simulink library "waijung_image_sensor_lib"  (R2015b)
settings: Solver=ode45  StartTime=0.0  StopTime=10.0  RelTol=1e-3
libraries: simulink x11, stm32f4_i2c_lib x8, stm32f4_tim_lib x2
settings Model: Creator=Krisada  LastModifiedBy=Aimagin
settings DataIOCC: SaveFormat=Array  SignalLoggingSaveFormat=ModelDataLogs
settings OptimizationCC: ExpressionDepthLimit=2147483647
settings DebuggingCC: UnderspecifiedInitializationDetection=Classic  MergeDetectMultiDrivingBlocksExec=none  SolverPrmCheckMsg=warning  FcnCallInpInsideContextMsg=UseLocalSettings  StateNameClashWarn=warning  StrictBusMsg=Warning
settings HardwareCC: ProdBitPerPointer=32  ProdLargestAtomicFloat=None  ProdIntDivRoundTo=Undefined  ProdEndianess=Unspecified  ProdWordSize=32  ProdHWDeviceType=32-bit Generic
settings GRTTargetCC: CombineOutputUpdateFcns=off  GRTInterface=on
settings ConfigComp: CovModelRefEnable=Off

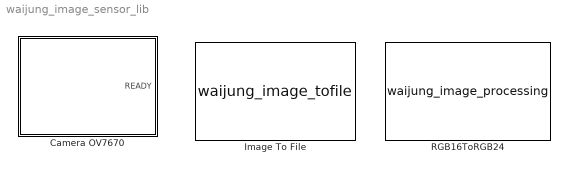
== system waijung_image_sensor_lib ==
  Camera OV7670 : Subsystem  mask{camera=OV7670, storagename=ExtRAM, xclkfreq=8MHz(MCO), imgsize=120 x 160, module=1, slvaddr=hex2dec('42'), sampletime=-1}
      mask prompts: storagename "Output buffer"; xclkfreq "XCLK input frequency"; imgsize "Image size"; module "I2C Module"; slvaddr "I2C Slave address"; sampletime "Sample time (sec)"
      mask init:
      | waijung_image_sensor_callback('init');
      mask TypeOptions camera: OV7670
      mask Callback camera: waijung_image_sensor_callback('camera');
      mask TypeOptions storagename: ExtRAM
      mask Callback storagename: waijung_image_sensor_callback('storagename');
      mask TypeOptions xclkfreq: 8MHz(MCO) | 24MHz
      mask TypeOptions imgsize: 120 x 160 | 240 x 320 | 480 x 640
      mask TypeOptions module: 1 | 2 | 3
      mask Callback module: waijung_image_sensor_callback('module');
      mask Display: text(0.5, 0.5, '[OV7670]\nPort: I2C1','ver','middle','hor','center');port_label('output', 1,'READY');
  Image To File : S-Function  FunctionName=waijung_image_tofile  Parameters=conf,inputporttype,inputportwidth,outputporttype,outputportwidth,optionstring,sampletime,blockid  SFunctionDeploymentMode=off  EnableBusSupport=off  mask(waijung_image_tofile){conf=ToFile, variablefilename=on, filename=Image.bmp, format=BMP, size=QQVGA (160 x 120), storagename=<Manual Configure>, varname=0x64000000, storagetype=uint16, storagesize=160*120*2, portpinstr=0, rgb16torgb24=on, enablestatus=on, sampletime=-1, blockid=ImageToFile, inputporttype=[7], inputportwidth=[], inputportlabel={'Filename'}, outputporttype=[7], outputportwidth=[], outputportlabel={'Status'}, compat=0, optionstring=[]}
      mask prompts: conf "Configuration"; variablefilename "Variable file name"; filename "File name"; storagename "Source buffer"; varname "Source buffer var name"; storagetype "Source buffer var type"; storagesize "Source buffer size"; portpinstr "Port Pin String"; rgb16torgb24 "Enable RGB16 to RGB24 conversion"; enablestatus "Enable output status"; sampletime "Sample time (sec)"; blockid "Block ID"; inputporttype "Input Port Type"; inputportwidth "Input Port Width"; inputportlabel "Input Port Label"; outputporttype "Output Port Type"; outputportwidth "Output Port Width"; outputportlabel "Output port label"; compat "Compatibility (Reserved for future use)"; optionstring "String(s) to be passed to TLC"
      mask init:
      | waijung_image_tofile_callback('init');
      mask Help: web(fullfile(waijungdocroot,'waijung_image_tofile.htm'), '-browser')
      mask TypeOptions conf: ToFile
      mask Callback conf: waijung_image_tofile_callback('conf');
      mask Callback variablefilename: waijung_image_tofile_callback('variablefilename');
      mask TypeOptions format: BMP | JPG
      mask TypeOptions size: QQVGA (160 x 120) | QVGA (320 x 240) | VGA (640 x 480)
      mask TypeOptions storagename: <Manual Configure>
      mask Callback storagename: stm32f4_dcmi_callback('storagename');
      mask TypeOptions storagetype: double | single | int8 | uint8 | int16 | uint16 | int32 | uint32
      mask Callback enablestatus: waijung_image_tofile_callback('enablestatus');
      mask Callback sampletime: waijung_image_tofile_callback('sampletime');
      mask Callback blockid: waijung_image_tofile_callback('blockid');
      mask Display: text(0.5, 0.5, '[ BMP ]\nQQVGA (160 x 120)','ver','middle','hor','center'); port_label('input', 1,'Filename'); port_label('output', 1,'Status');
  RGB16ToRGB24 : S-Function  FunctionName=waijung_image_processing  Parameters=conf,inputporttype,inputportwidth,outputporttype,outputportwidth,row,column,optionstring,simparams,sampletime,blockid  SFunctionDeploymentMode=off  EnableBusSupport=off  mask(waijung_image_processing){conf=RGB16ToRGB24, column=10, row=10, inputalignment=RGB, outputalignment=RGB, colorseparate=on, simparams=[0 10 0 0], portpinstr=0, sampletime=-1, blockid=RGB16ToRGB24, inputporttype=[5], inputportwidth=[100], inputportlabel={'Input'}, outputporttype=[3  3 3], outputportwidth=[10 10 10], outputportlabel={'R','G','B'}, compat=0, optionstring=[]}
      mask prompts: conf "Configuration"; column "Image width (Column, M)"; row "Image heigh (Row, N)"; inputalignment "Input color alignment"; outputalignment "Output color alignment"; colorseparate "Separate output color"; simparams "Simulate params"; portpinstr "Port Pin String"; sampletime "Sample time (sec)"; blockid "Block ID"; inputporttype "Input Port Type"; inputportwidth "Input Port Width"; inputportlabel "Input Port Label"; outputporttype "Output Port Type"; outputportwidth "Output Port Width"; outputportlabel "Output port label"; compat "Compatibility (Reserved for future use)"; optionstring "String(s) to be passed to TLC"
      mask help: RGB16: R(5)-G(6)-B(5)
      mask init:
      | waijung_image_processing_callback('init');
      mask Help: web(fullfile(waijungdocroot,'waijung_image_processing.htm'), '-browser')
      mask TypeOptions conf: RGB16ToRGB24
      mask Callback conf: waijung_image_processing_callback('conf');
      mask Callback column: waijung_image_processing_callback('updateport');
      mask TypeOptions inputalignment: RGB | BGR
      mask Callback inputalignment: waijung_image_processing_callback('updateport');
      mask TypeOptions outputalignment: RGB | BGR
      mask Callback outputalignment: waijung_image_processing_callback('updateport');
      mask Callback colorseparate: waijung_image_processing_callback('updateport');
      mask Callback sampletime: waijung_image_processing_callback('sampletime');
      mask Callback blockid: waijung_image_processing_callback('blockid');
      mask Display: text(0.5, 0.5, '[RGB16ToRGB24]','ver','middle','hor','center'); port_label('input', 1,'Input'); port_label('output', 1,'R'); port_label('output', 2,'G'); port_label('output', 3,'B');

== system waijung_image_sensor_lib/Camera OV7670 ==
  Capture_ : Subsystem  TreatAsAtomicUnit=on
  Init_ : Subsystem
  Logical Operator : Logic  Operator=NOT  AllPortsSameDT=off  OutDataTypeStr=boolean
  Memory : Memory  InheritSampleTime=on
  Rate Transition : RateTransition  OutPortSampleTime=sampletime
  READY : Outport
  wires:
  Capture_/1(SUCCESS) -> READY/1
  Init_/1(Out1) -> Memory/1
  Memory/1 -> Logical Operator/1, Rate Transition/1
  Logical Operator/1 -> Init_/Enable
  Rate Transition/1 -> Capture_/Enable

== system waijung_image_sensor_lib/Camera OV7670/Capture_ ==
  Enable : EnablePort  PropagateVarSize=During execution
  Compare To Zero : simulink/Logic and Bit Operations/Compare To Zero  SystemSampleTime=-1  relop===  LogicOutDataTypeMode=uint8  ZeroCross=off
  DCMI Capture : S-Function  FunctionName=stm32f4_dcmi  Parameters=conf,inputporttype,inputportwidth,outputporttype,outputportwidth,optionstring,sampletime,blockid  SFunctionDeploymentMode=off  EnableBusSupport=off  mask(stm32f4_dcmi){conf=DCMI, capturemode=SnapShot, synchronizemode=Hardware, pclkpolarity=Falling, vspolarity=High, hspolarity=High, capturerate=All, capturesize=120*160*2, storagename=<Manual Configure>, varname=VolatileDataArray_ExtRAM, storagetype=uint16, storagesize=120*160, remap=Profile #2, sampletime=inf, blockid=CameraOV7670Capture_DCMICapture, inputporttype=[], inputportwidth=[], inputportlabel={}, outputporttype=[7], outputportwidth=[], outputportlabel={'Status'}, compat=0, optionstring=["DCMI","SnapShot","Hardware","Falling","High","High","All","0","Word","9600","0","0","VolatileDataArray_ExtRAM"," "," "," ","1","0","0","0","0","0","0","1","1","A","6","I","5","H","8","H","9","H","10","H","11","H","12","H","14","I","4","I","6","I","7"], portpinstr=A6,I5,H8,H9,H10,H11,H12,H14,I4,I6,I7}
      mask prompts: conf "Configuration"; capturemode "Capture mode"; synchronizemode "Synchronization Mode"; pclkpolarity "Pixel clock polarity"; vspolarity "Vertical synchronization polarity"; hspolarity "Horizontal synchronization polarity"; capturerate "Capture rate"; capturesize "Capture data size (Bytes)"; storagename "Output buffer"; varname "Output buffer var name"; storagetype "Output buffer var type"; storagesize "Output buffer size (Total bytes must be equal to, or greater than DMA Transfer size)"; remap "Remap DCMI pins"; sampletime "Sample time (sec)"; inputporttype "Input port"; inputportwidth "Input Port Width"; inputportlabel "Input port label"; outputporttype "Output port"; outputportwidth "Output Port Width"; outputportlabel "Output port label"; compat "Compatibility (Reserved for future use)"; optionstring "Configuration String"; portpinstr "Port Pin String"
      mask help:
      | Synchronize mode:
      |  - Hardware: Hardware synchronization data capture is synchronized with the HSYNC/VSYNC signals.
      |  - Embedded: Embedded synchronization data capture is synchronized with synchronization codes embedded in the data flow.
      | Pixel clock polarity:
      |  - Falling: Pixel clock active on Falling edge.
      |  - Rising: Pixel clock active on Rising edge.
      | Vertical, Horizontal sychronization polarity:
      |  - Low: vertical synchronization active Low.
      |  - High: Vertical synchronization active High.
      | Capture rate:
      |  - All: All frames are captured.
      |  - 1of2: Every alternate frame captured.
      |  - 1of4: On frame in 4 frames captured.
      | Pins Profile:
      | Set of configuration pins for: PIXCLK, VSYNC, HSYNC, D0, D1, .., D7 corresponding.
      |  - Profile #1: PA6, PB7, PA4, PC6, PC7,  PE0,  PE1,  PE4,  PB6, PE5, PE6
      |  - Profile #2: PA6, PI5, PH8, PH9, PH10, PH11, PH12, PH14, PI4, PI6, PI7
      mask init:
      | stm32f4_dcmi_callback('init');
      mask Help: web(fullfile(waijungdocroot,'stm32f4_dcmi.htm'), '-browser')
      mask TypeOptions conf: DCMI
      mask Callback conf: stm32f4_dcmi_callback('conf');
      mask TypeOptions capturemode: Continuous | SnapShot
      mask TypeOptions synchronizemode: Hardware | Embedded
      mask TypeOptions pclkpolarity: Falling | Rising
      mask TypeOptions vspolarity: High | Low
      mask TypeOptions hspolarity: High | Low
      mask TypeOptions capturerate: All | 1of2 | 1of4
      mask TypeOptions storagename: <Manual Configure>
      mask Callback storagename: stm32f4_dcmi_callback('storagename');
      mask TypeOptions storagetype: double | single | int8 | uint8 | int16 | uint16 | int32 | uint32
      mask Callback storagesize: stm32f4_dcmi_callback('storagesize');
      mask TypeOptions remap: Profile #1 | Profile #2
      mask Callback remap: stm32f4_dcmi_callback('remap');
      mask Callback sampletime: stm32f4_dcmi_callback('sampletime');
      mask Callback blockid: stm32f4_dcmi_callback('blockid');
      mask Display: text(0.05, 0.5, 'Size: 38400\nPins: Profile #2\nTs (sec): 0','ver','middle','hor','left'); port_label('output', 1,'Status');
  SUCCESS : Outport
  wires:
  Compare To Zero/1 -> SUCCESS/1
  DCMI Capture/1 -> Compare To Zero/1

== system waijung_image_sensor_lib/Camera OV7670/Init_ ==
  Enable : EnablePort  PropagateVarSize=During execution
  While Iterator_ : Subsystem  TreatAsAtomicUnit=on
  Out1 : Outport
  wires:
  While Iterator_/1(Ready) -> Out1/1

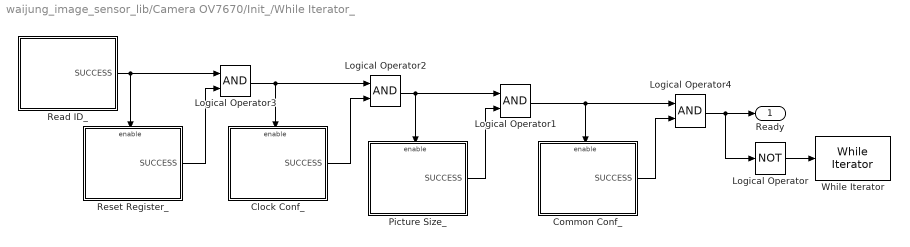
== system waijung_image_sensor_lib/Camera OV7670/Init_/While Iterator_ ==
  Clock Conf_ : Subsystem
  Common Conf_ : Subsystem
  Logical Operator : Logic  Operator=NOT  AllPortsSameDT=off  OutDataTypeStr=boolean
  Logical Operator{1..4} (4 alike) : Logic  AllPortsSameDT=off  OutDataTypeStr=boolean
  Picture Size_ : Subsystem
  Read ID_ : Subsystem
  Reset Register_ : Subsystem
  While Iterator : WhileIterator  MaxIters=-1  WhileBlockType=do-while
  Ready : Outport
  wires:
  Logical Operator3/1 -> Clock Conf_/Enable, Logical Operator2/1
  Read ID_/1(SUCCESS) -> Reset Register_/Enable, Logical Operator3/1
  Picture Size_/1(SUCCESS) -> Logical Operator1/2
  Logical Operator1/1 -> Common Conf_/Enable, Logical Operator4/1
  Logical Operator/1 -> While Iterator/1
  Reset Register_/1(SUCCESS) -> Logical Operator3/2
  Clock Conf_/1(SUCCESS) -> Logical Operator2/2
  Logical Operator2/1 -> Logical Operator1/1, Picture Size_/Enable
  Logical Operator4/1 -> Logical Operator/1, Ready/1
  Common Conf_/1(SUCCESS) -> Logical Operator4/2

== system waijung_image_sensor_lib/Camera OV7670/Init_/While Iterator_/Clock Conf_ ==
  Enable : EnablePort  PropagateVarSize=During execution
  Logical Operator : Logic  Operator=NOT  AllPortsSameDT=off  OutDataTypeStr=boolean
  Memory : Memory  InheritSampleTime=on
  Subsystem : Subsystem
  SUCCESS : Outport
  wires:
  Memory/1 -> Logical Operator/1
  Logical Operator/1 -> Subsystem/Enable
  Subsystem/1(Out1) -> Memory/1, SUCCESS/1

== system waijung_image_sensor_lib/Camera OV7670/Init_/While Iterator_/Common Conf_ ==
  Enable : EnablePort  PropagateVarSize=During execution
  Logical Operator : Logic  Operator=NOT  AllPortsSameDT=off  OutDataTypeStr=boolean
  Memory : Memory  InheritSampleTime=on
  Subsystem : Subsystem
  SUCCESS : Outport
  wires:
  Memory/1 -> Logical Operator/1
  Logical Operator/1 -> Subsystem/Enable
  Subsystem/1(Out1) -> Memory/1, SUCCESS/1

== system waijung_image_sensor_lib/Camera OV7670/Init_/While Iterator_/Picture Size_ ==
  Enable : EnablePort  PropagateVarSize=During execution
  Logical Operator : Logic  Operator=NOT  AllPortsSameDT=off  OutDataTypeStr=boolean
  Memory : Memory  InheritSampleTime=on
  Subsystem : Subsystem
  SUCCESS : Outport
  wires:
  Subsystem/1(Out1) -> SUCCESS/1, Memory/1
  Logical Operator/1 -> Subsystem/Enable
  Memory/1 -> Logical Operator/1

== system waijung_image_sensor_lib/Camera OV7670/Init_/While Iterator_/Read ID_ ==
  Logical Operator : Logic  Operator=NOT  AllPortsSameDT=off  OutDataTypeStr=boolean
  Memory : Memory  InheritSampleTime=on
  Subsystem_ : Subsystem
  SUCCESS : Outport
  wires:
  Subsystem_/1(Out1) -> SUCCESS/1, Memory/1
  Logical Operator/1 -> Subsystem_/Enable
  Memory/1 -> Logical Operator/1

== system waijung_image_sensor_lib/Camera OV7670/Init_/While Iterator_/Reset Register_ ==
  Enable : EnablePort  PropagateVarSize=During execution
  Logical Operator : Logic  Operator=NOT  AllPortsSameDT=off  OutDataTypeStr=boolean
  Memory : Memory  InheritSampleTime=on
  Subsystem : Subsystem
  SUCCESS : Outport
  wires:
  Memory/1 -> Logical Operator/1
  Logical Operator/1 -> Subsystem/Enable
  Subsystem/1(Out1) -> Memory/1, SUCCESS/1

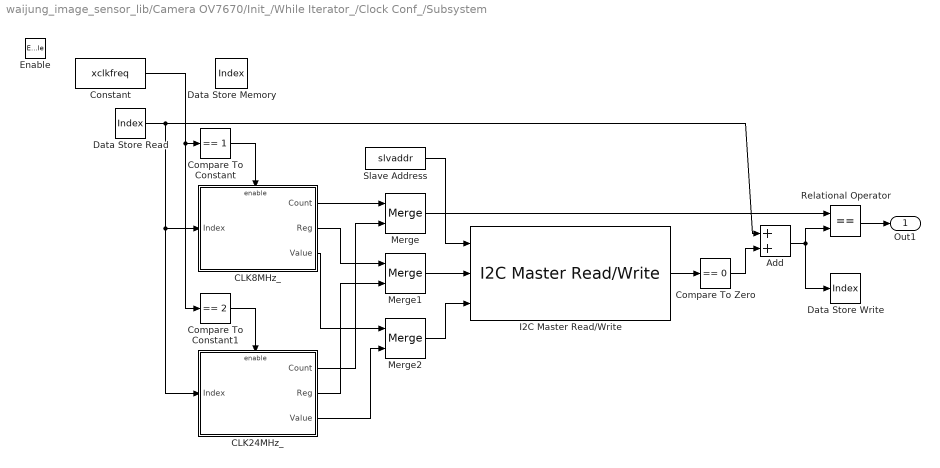
== system waijung_image_sensor_lib/Camera OV7670/Init_/While Iterator_/Clock Conf_/Subsystem ==
  Enable : EnablePort  PropagateVarSize=During execution
  Add : Sum
  CLK24MHz_ : Subsystem  TreatAsAtomicUnit=on
  CLK8MHz_ : Subsystem  TreatAsAtomicUnit=on
  Compare To Constant : simulink/Logic and Bit Operations/Compare To Constant  SystemSampleTime=-1  relop===  const=1  LogicOutDataTypeMode=boolean  ZeroCross=off
  Compare To Constant1 : simulink/Logic and Bit Operations/Compare To Constant  SystemSampleTime=-1  relop===  const=2  LogicOutDataTypeMode=boolean  ZeroCross=off
  Compare To Zero : simulink/Logic and Bit Operations/Compare To Zero  SystemSampleTime=-1  relop===  LogicOutDataTypeMode=uint8  ZeroCross=off
  Constant : Constant  Value=xclkfreq
  Data Store Memory : DataStoreMemory  DataStoreName=Index  ReadBeforeWriteMsg=warning  WriteAfterWriteMsg=warning  WriteAfterReadMsg=warning  OutDataTypeStr=uint8
  Data Store Read : DataStoreRead  DataStoreName=Index
  Data Store Write : DataStoreWrite  DataStoreName=Index
  I2C Master Read/Write : stm32f4_i2c_lib/I2C Master Read//Write  configuration=Transaction  module=1  lastmodule=3  transfer=Blocking  dutycycle=TLow/THigh = 2  clkspeed=400  timeout=25  writecount=2  readcount=0  sdapin=C9  sclpin=A8  waitwritetime=5  forcestop=off  inputtypearray=[3 3 3 3]  outputtypearray=[1 3]  confstr="[\"C\",\"9\",\"A\",\"8\",\"1\",\"1\",\"6\",\"0\",\"I2C_DutyCycle_2\",\"5\",\"off\"]"  sampletime=-1  sampletimestr=-1  blockid=CameraOV1Init_WhileIterator_ClockConf_SubsystemI2CMasterReadWrite
  Merge : Merge
  Merge1 : Merge
  Merge2 : Merge
  Relational Operator : RelationalOperator  Operator===  OutDataTypeStr=boolean
  Slave Address : Constant  Value=slvaddr  OutDataTypeStr=uint8
  Out1 : Outport
  wires:
  Relational Operator/1 -> Out1/1
  Add/1 -> Data Store Write/1, Relational Operator/2
  Compare To Zero/1 -> Add/2
  I2C Master Read/Write/1 -> Compare To Zero/1
  Data Store Read/1 -> Add/1, CLK8MHz_/1(Index), CLK24MHz_/1(Index)
  Slave Address/1 -> I2C Master Read/Write/1
  Compare To Constant/1 -> CLK8MHz_/Enable
  Compare To Constant1/1 -> CLK24MHz_/Enable
  CLK8MHz_/1(Count) -> Merge/1
  CLK8MHz_/2(Reg) -> Merge1/1
  CLK8MHz_/3(Value) -> Merge2/1
  CLK24MHz_/1(Count) -> Merge/2
  CLK24MHz_/2(Reg) -> Merge1/2
  CLK24MHz_/3(Value) -> Merge2/2
  Constant/1 -> Compare To Constant/1, Compare To Constant1/1
  Merge/1 -> Relational Operator/1
  Merge1/1 -> I2C Master Read/Write/2
  Merge2/1 -> I2C Master Read/Write/3

== system waijung_image_sensor_lib/Camera OV7670/Init_/While Iterator_/Common Conf_/Subsystem ==
  Enable : EnablePort  PropagateVarSize=During execution
  Add : Sum
  Compare To Zero : simulink/Logic and Bit Operations/Compare To Zero  SystemSampleTime=-1  relop===  LogicOutDataTypeMode=uint8  ZeroCross=off
  Data Store Memory : DataStoreMemory  DataStoreName=Index  ReadBeforeWriteMsg=warning  WriteAfterWriteMsg=warning  WriteAfterReadMsg=warning  OutDataTypeStr=uint8
  Data Store Read : DataStoreRead  DataStoreName=Index
  Data Store Write : DataStoreWrite  DataStoreName=Index
  I2C Master Read/Write : stm32f4_i2c_lib/I2C Master Read//Write  configuration=Transaction  module=1  lastmodule=3  transfer=Blocking  dutycycle=TLow/THigh = 2  clkspeed=400  timeout=25  writecount=2  readcount=0  sdapin=C9  sclpin=A8  waitwritetime=5  forcestop=off  inputtypearray=[3 3 3 3]  outputtypearray=[1 3]  confstr="[\"C\",\"9\",\"A\",\"8\",\"1\",\"1\",\"6\",\"0\",\"I2C_DutyCycle_2\",\"5\",\"off\"]"  sampletime=-1  sampletimestr=-1  blockid=CameraOV1Init_WhileIterator_CommonConf_SubsystemI2CMasterReadWrite
  Register List : Subsystem  mask{register=uint8([122,123,124,125,126,127,128,129,130,131,132,133,134,135,136,137,19,21,0,16,13,20,165,171,36,37,38,159,160,161,166,167,168,169,170,19,14,15,22,30,33,34,41,51,53,55,56,57,60,77,78,105,116,141,142,143,144,145,146,150,154,176,177,178,179,184,67,68,69,70,71,72,89,90,91,92,93,94,100,101,102,148,149,108,109,110,111,106,1,2,19,21,79,80,81,82,83,84,85,86,87,88,65,63,117,118,76,119,75,201,65,86,52,59,164,150,157,158,9,59]), value=uint8([32,28,40,60,85,104,118,128,136,143,150,163,175,196,215,232,232,24,15,0,0,32,5,7,117,99,165,120,104,3,223,223,240,144,148,229,97,75,2,39,2,145,7,11,11,29,113,42,120,64,32,0,25,79,0,0,0,0,0,0,128,132,12,14,130,10,20,240,52,88,40,58,136,136,68,103,73,14,4,32,5,4,8,10,85,17,159,64,64,64,231,24,128,128,0,34,94,128,0,82,128,158,8,5,5,225,15,10,9,192,56,64,17,2,137,0,76,63,2,66])}
      mask prompts: register "Register Index"; value "Register Value"
      mask help:
      | Count:
      |  - Number of Register-Value pair.
      |  - Determine from lowest size, between Register and Value.
      | Reg:
      |  - Register index.
      | Value:
      |  - Data corresponding to specified register index.
  Relational Operator : RelationalOperator  Operator===  OutDataTypeStr=boolean
  Slave Address : Constant  Value=slvaddr  OutDataTypeStr=uint8
  Out1 : Outport
  wires:
  Register List/1(Count) -> Relational Operator/1
  Register List/3(Value) -> I2C Master Read/Write/3
  Register List/2(Reg) -> I2C Master Read/Write/2
  Relational Operator/1 -> Out1/1
  Add/1 -> Data Store Write/1, Relational Operator/2
  Compare To Zero/1 -> Add/2
  I2C Master Read/Write/1 -> Compare To Zero/1
  Data Store Read/1 -> Register List/1(Index), Add/1
  Slave Address/1 -> I2C Master Read/Write/1

== system waijung_image_sensor_lib/Camera OV7670/Init_/While Iterator_/Picture Size_/Subsystem ==
  Enable : EnablePort  PropagateVarSize=During execution
  Add : Sum
  Compare To Zero : simulink/Logic and Bit Operations/Compare To Zero  SystemSampleTime=-1  relop===  LogicOutDataTypeMode=uint8  ZeroCross=off
  Data Store Memory : DataStoreMemory  DataStoreName=Index  ReadBeforeWriteMsg=warning  WriteAfterWriteMsg=warning  WriteAfterReadMsg=warning  OutDataTypeStr=uint8
  Data Store Read : DataStoreRead  DataStoreName=Index
  Data Store Write : DataStoreWrite  DataStoreName=Index
  I2C Master Read/Write : stm32f4_i2c_lib/I2C Master Read//Write  configuration=Transaction  module=1  lastmodule=3  transfer=Blocking  dutycycle=TLow/THigh = 2  clkspeed=400  timeout=25  writecount=2  readcount=0  sdapin=C9  sclpin=A8  waitwritetime=5  forcestop=off  inputtypearray=[3 3 3 3]  outputtypearray=[1 3]  confstr="[\"C\",\"9\",\"A\",\"8\",\"1\",\"1\",\"6\",\"0\",\"I2C_DutyCycle_2\",\"5\",\"off\"]"  sampletime=-1  sampletimestr=-1  blockid=CameraOV1Init_WhileIterator_PictureSize_SubsystemI2CMasterReadWrite
  Relational Operator : RelationalOperator  Operator===  OutDataTypeStr=boolean
  Slave Address : Constant  Value=slvaddr  OutDataTypeStr=uint8
  Subsystem : Subsystem
  Out1 : Outport
  wires:
  Slave Address/1 -> I2C Master Read/Write/1
  Data Store Read/1 -> Add/1, Subsystem/1(Index)
  I2C Master Read/Write/1 -> Compare To Zero/1
  Compare To Zero/1 -> Add/2
  Add/1 -> Relational Operator/2, Data Store Write/1
  Relational Operator/1 -> Out1/1
  Subsystem/3(Value) -> I2C Master Read/Write/3
  Subsystem/2(Reg) -> I2C Master Read/Write/2
  Subsystem/1(Count) -> Relational Operator/1

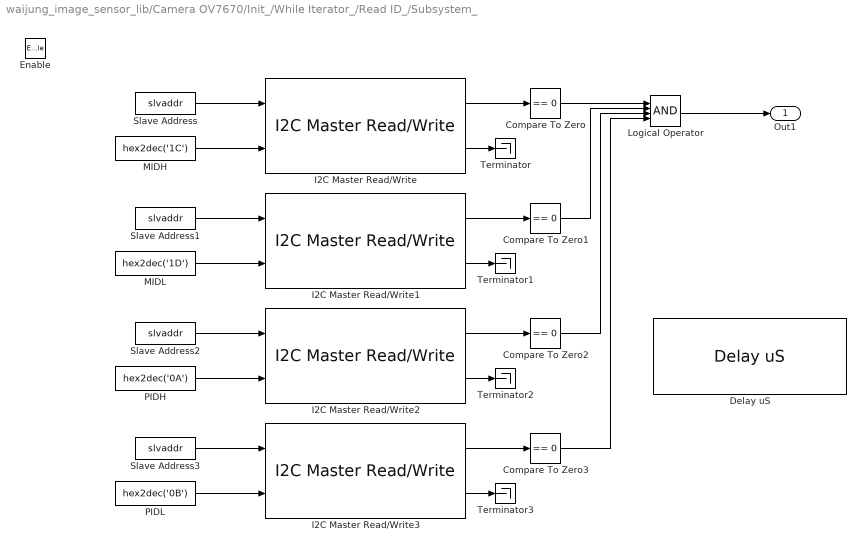
== system waijung_image_sensor_lib/Camera OV7670/Init_/While Iterator_/Read ID_/Subsystem_ ==
  Enable : EnablePort  PropagateVarSize=During execution
  Compare To Zero{,1..3} (4 alike) : simulink/Logic and Bit Operations/Compare To Zero  SystemSampleTime=-1  relop===  LogicOutDataTypeMode=uint8  ZeroCross=off
  Delay uS : stm32f4_tim_lib/Delay uS  Priority=0  delaytime=300000  enableinput=off  enableoutput=off  inputtypearray=[0]  outputtypearray=[0]  sampletime=-1  sampletimestr=-1  blockid=CameraOV1Init_WhileIterator_ReadID_Subsystem_DelayuS
  I2C Master Read/Write : stm32f4_i2c_lib/I2C Master Read//Write  configuration=Transaction  module=1  lastmodule=3  transfer=Blocking  dutycycle=TLow/THigh = 2  clkspeed=400  timeout=25  writecount=1  readcount=1  sdapin=C9  sclpin=A8  waitwritetime=0  forcestop=on  inputtypearray=[2 3 3]  outputtypearray=[2 3 3]  confstr="[\"C\",\"9\",\"A\",\"8\",\"1\",\"1\",\"6\",\"0\",\"I2C_DutyCycle_2\",\"0\",\"on\"]"  sampletime=-1  sampletimestr=-1  blockid=CameraOV1Init_WhileIterator_ReadID_Subsystem_I2CMasterReadWrite
  I2C Master Read/Write1 : stm32f4_i2c_lib/I2C Master Read//Write  configuration=Transaction  module=1  lastmodule=3  transfer=Blocking  dutycycle=TLow/THigh = 2  clkspeed=400  timeout=25  writecount=1  readcount=1  sdapin=C9  sclpin=A8  waitwritetime=0  forcestop=on  inputtypearray=[2 3 3]  outputtypearray=[2 3 3]  confstr="[\"C\",\"9\",\"A\",\"8\",\"1\",\"1\",\"6\",\"0\",\"I2C_DutyCycle_2\",\"0\",\"on\"]"  sampletime=-1  sampletimestr=-1  blockid=CameraOV1Init_WhileIterator_ReadID_Subsystem_I2CMasterReadWrite1
  I2C Master Read/Write2 : stm32f4_i2c_lib/I2C Master Read//Write  configuration=Transaction  module=1  lastmodule=3  transfer=Blocking  dutycycle=TLow/THigh = 2  clkspeed=400  timeout=25  writecount=1  readcount=1  sdapin=C9  sclpin=A8  waitwritetime=0  forcestop=on  inputtypearray=[2 3 3]  outputtypearray=[2 3 3]  confstr="[\"C\",\"9\",\"A\",\"8\",\"1\",\"1\",\"6\",\"0\",\"I2C_DutyCycle_2\",\"0\",\"on\"]"  sampletime=-1  sampletimestr=-1  blockid=CameraOV1Init_WhileIterator_ReadID_Subsystem_I2CMasterReadWrite2
  I2C Master Read/Write3 : stm32f4_i2c_lib/I2C Master Read//Write  configuration=Transaction  module=1  lastmodule=3  transfer=Blocking  dutycycle=TLow/THigh = 2  clkspeed=400  timeout=25  writecount=1  readcount=1  sdapin=C9  sclpin=A8  waitwritetime=0  forcestop=on  inputtypearray=[2 3 3]  outputtypearray=[2 3 3]  confstr="[\"C\",\"9\",\"A\",\"8\",\"1\",\"1\",\"6\",\"0\",\"I2C_DutyCycle_2\",\"0\",\"on\"]"  sampletime=-1  sampletimestr=-1  blockid=CameraOV1Init_WhileIterator_ReadID_Subsystem_I2CMasterReadWrite3
  Logical Operator : Logic  Inputs=4  AllPortsSameDT=off  OutDataTypeStr=boolean
  MIDH : Constant  Value=hex2dec('1C')  OutDataTypeStr=uint8
  MIDL : Constant  Value=hex2dec('1D')  OutDataTypeStr=uint8
  PIDH : Constant  Value=hex2dec('0A')  OutDataTypeStr=uint8
  PIDL : Constant  Value=hex2dec('0B')  OutDataTypeStr=uint8
  Slave Address{,1..3} (4 alike) : Constant  Value=slvaddr  OutDataTypeStr=uint8
  Terminator{,1..3} (4 alike) : Terminator
  Out1 : Outport
  wires:
  Slave Address/1 -> I2C Master Read/Write/1
  MIDH/1 -> I2C Master Read/Write/2
  Slave Address1/1 -> I2C Master Read/Write1/1
  MIDL/1 -> I2C Master Read/Write1/2
  Slave Address2/1 -> I2C Master Read/Write2/1
  PIDH/1 -> I2C Master Read/Write2/2
  Slave Address3/1 -> I2C Master Read/Write3/1
  PIDL/1 -> I2C Master Read/Write3/2
  I2C Master Read/Write/1 -> Compare To Zero/1
  I2C Master Read/Write1/1 -> Compare To Zero1/1
  I2C Master Read/Write2/1 -> Compare To Zero2/1
  I2C Master Read/Write3/1 -> Compare To Zero3/1
  Compare To Zero/1 -> Logical Operator/1
  Compare To Zero1/1 -> Logical Operator/2
  Compare To Zero3/1 -> Logical Operator/4
  Compare To Zero2/1 -> Logical Operator/3
  Logical Operator/1 -> Out1/1
  I2C Master Read/Write/2 -> Terminator/1
  I2C Master Read/Write1/2 -> Terminator1/1
  I2C Master Read/Write2/2 -> Terminator2/1
  I2C Master Read/Write3/2 -> Terminator3/1

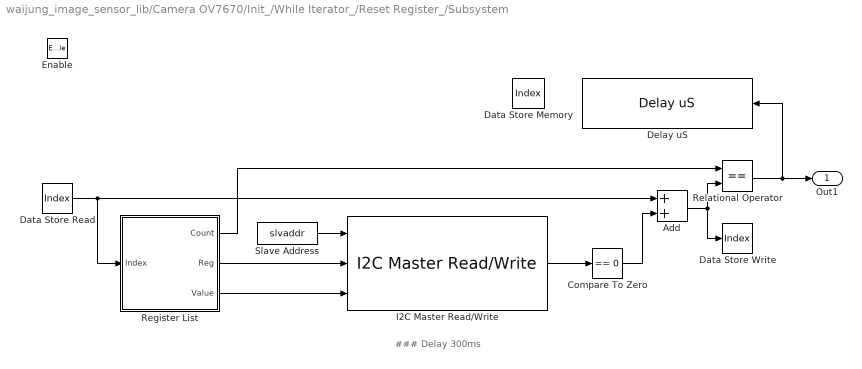
== system waijung_image_sensor_lib/Camera OV7670/Init_/While Iterator_/Reset Register_/Subsystem ==
  note: ### Delay 300ms
  Enable : EnablePort  PropagateVarSize=During execution
  Add : Sum
  Compare To Zero : simulink/Logic and Bit Operations/Compare To Zero  SystemSampleTime=-1  relop===  LogicOutDataTypeMode=uint8  ZeroCross=off
  Data Store Memory : DataStoreMemory  DataStoreName=Index  ReadBeforeWriteMsg=warning  WriteAfterWriteMsg=warning  WriteAfterReadMsg=warning  OutDataTypeStr=uint8
  Data Store Read : DataStoreRead  DataStoreName=Index
  Data Store Write : DataStoreWrite  DataStoreName=Index
  Delay uS : stm32f4_tim_lib/Delay uS  delaytime=200000  enableinput=on  enableoutput=off  inputtypearray=[1 -1]  outputtypearray=[0]  sampletime=-1  sampletimestr=-1  blockid=CameraOV1Init_WhileIterator_ResetRegister_SubsystemDelayuS
  I2C Master Read/Write : stm32f4_i2c_lib/I2C Master Read//Write  configuration=Transaction  module=1  lastmodule=3  transfer=Blocking  dutycycle=TLow/THigh = 2  clkspeed=400  timeout=25  writecount=2  readcount=0  sdapin=C9  sclpin=A8  waitwritetime=300  forcestop=off  inputtypearray=[3 3 3 3]  outputtypearray=[1 3]  confstr="[\"C\",\"9\",\"A\",\"8\",\"1\",\"1\",\"6\",\"0\",\"I2C_DutyCycle_2\",\"300\",\"off\"]"  sampletime=-1  sampletimestr=-1  blockid=CameraOV1Init_WhileIterator_ResetRegister_SubsystemI2CMasterReadWrite
  Register List : Subsystem  mask{register=uint8([hex2dec('12')]), value=uint8([hex2dec('80')])}
      mask prompts: register "Register Index"; value "Register Value"
      mask help:
      | Count:
      |  - Number of Register-Value pair.
      |  - Determine from lowest size, between Register and Value.
      | Reg:
      |  - Register index.
      | Value:
      |  - Data corresponding to specified register index.
  Relational Operator : RelationalOperator  Operator===  OutDataTypeStr=boolean
  Slave Address : Constant  Value=slvaddr  OutDataTypeStr=uint8
  Out1 : Outport
  wires:
  Register List/1(Count) -> Relational Operator/1
  Register List/3(Value) -> I2C Master Read/Write/3
  Register List/2(Reg) -> I2C Master Read/Write/2
  Relational Operator/1 -> Out1/1, Delay uS/1
  Add/1 -> Data Store Write/1, Relational Operator/2
  Compare To Zero/1 -> Add/2
  I2C Master Read/Write/1 -> Compare To Zero/1
  Data Store Read/1 -> Register List/1(Index), Add/1
  Slave Address/1 -> I2C Master Read/Write/1

== system waijung_image_sensor_lib/Camera OV7670/Init_/While Iterator_/Clock Conf_/Subsystem/CLK24MHz_ ==
  Index : Inport
  Enable : EnablePort  PropagateVarSize=During execution
  Reg List_ : Subsystem  mask{register=uint8([17 107]), value=uint8([1 74])}
      mask prompts: register "Register Index"; value "Register Value"
      mask help:
      | Count:
      |  - Number of Register-Value pair.
      |  - Determine from lowest size, between Register and Value.
      | Reg:
      |  - Register index.
      | Value:
      |  - Data corresponding to specified register index.
  Count : Outport
  Reg : Outport  Port=2
  Value : Outport  Port=3
  wires:
  Index/1 -> Reg List_/1(Index)
  Reg List_/3(Value) -> Value/1
  Reg List_/2(Reg) -> Reg/1
  Reg List_/1(Count) -> Count/1

== system waijung_image_sensor_lib/Camera OV7670/Init_/While Iterator_/Clock Conf_/Subsystem/CLK8MHz_ ==
  Index : Inport
  Enable : EnablePort  PropagateVarSize=During execution
  Reg List_ : Subsystem  mask{register=uint8([hex2dec('11') hex2dec('6B')]), value=uint8([hex2dec('00') hex2dec('80')])}
      mask prompts: register "Register Index"; value "Register Value"
      mask help:
      | Count:
      |  - Number of Register-Value pair.
      |  - Determine from lowest size, between Register and Value.
      | Reg:
      |  - Register index.
      | Value:
      |  - Data corresponding to specified register index.
  Count : Outport
  Reg : Outport  Port=2
  Value : Outport  Port=3
  wires:
  Reg List_/1(Count) -> Count/1
  Reg List_/2(Reg) -> Reg/1
  Reg List_/3(Value) -> Value/1
  Index/1 -> Reg List_/1(Index)

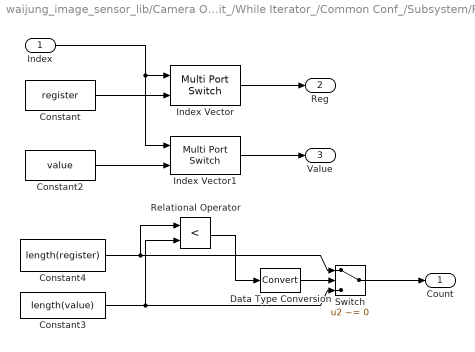
== system waijung_image_sensor_lib/Camera OV7670/Init_/While Iterator_/Common Conf_/Subsystem/Register List ==
  Index : Inport
  Constant : Constant  Value=register
  Constant2 : Constant  Value=value
  Constant3 : Constant  Value=length(value)
  Constant4 : Constant  Value=length(register)
  Data Type Conversion : DataTypeConversion
  Index Vector : MultiPortSwitch  DataPortOrder=Zero-based contiguous  Inputs=1  zeroidx=on
  Index Vector1 : MultiPortSwitch  DataPortOrder=Zero-based contiguous  Inputs=1  zeroidx=on
  Relational Operator : RelationalOperator  Operator=<  OutDataTypeStr=boolean
  Switch : Switch  Criteria=u2 ~= 0
  Count : Outport
  Reg : Outport  Port=2
  Value : Outport  Port=3
  wires:
  Index Vector/1 -> Reg/1
  Constant/1 -> Index Vector/2
  Index/1 -> Index Vector/1, Index Vector1/1
  Constant2/1 -> Index Vector1/2
  Index Vector1/1 -> Value/1
  Constant4/1 -> Relational Operator/1, Switch/1
  Constant3/1 -> Relational Operator/2, Switch/3
  Relational Operator/1 -> Data Type Conversion/1
  Switch/1 -> Count/1
  Data Type Conversion/1 -> Switch/2

== system waijung_image_sensor_lib/Camera OV7670/Init_/While Iterator_/Picture Size_/Subsystem/Subsystem ==
  Index : Inport
  Constant : Constant  Value=imgsize
  Img120x160 : Subsystem  TreatAsAtomicUnit=on
  Img240x320 : Subsystem  TreatAsAtomicUnit=on
  Img480x640 : Subsystem  TreatAsAtomicUnit=on
  Merge_Count : Merge  Inputs=3
  Merge_Reg : Merge  Inputs=3
  Merge_Value : Merge  Inputs=3
  Switch Case : SwitchCase  CaseConditions={1,2}
  Count : Outport
  Reg : Outport  Port=2
  Value : Outport  Port=3
  wires:
  Switch Case/1 -> Img120x160/Action
  Switch Case/2 -> Img240x320/Action
  Img120x160/1(Count) -> Merge_Count/1
  Img480x640/1(Count) -> Merge_Count/3
  Img240x320/1(Count) -> Merge_Count/2
  Img120x160/2(Reg) -> Merge_Reg/1
  Img240x320/2(Reg) -> Merge_Reg/2
  Img480x640/2(Reg) -> Merge_Reg/3
  Img120x160/3(Value) -> Merge_Value/1
  Img240x320/3(Value) -> Merge_Value/2
  Img480x640/3(Value) -> Merge_Value/3
  Index/1 -> Img120x160/1(Index), Img240x320/1(Index), Img480x640/1(Index)
  Merge_Count/1 -> Count/1
  Merge_Reg/1 -> Reg/1
  Merge_Value/1 -> Value/1
  Constant/1 -> Switch Case/1
  Switch Case/3 -> Img480x640/Action

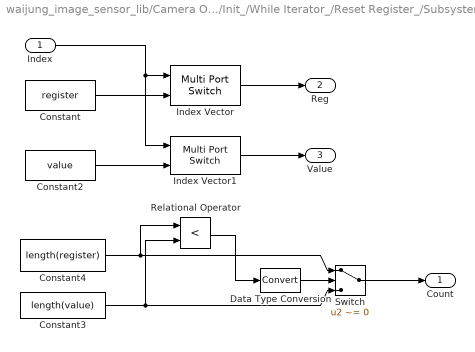
== system waijung_image_sensor_lib/Camera OV7670/Init_/While Iterator_/Reset Register_/Subsystem/Register List ==
  Index : Inport
  Constant : Constant  Value=register
  Constant2 : Constant  Value=value
  Constant3 : Constant  Value=length(value)
  Constant4 : Constant  Value=length(register)
  Data Type Conversion : DataTypeConversion
  Index Vector : MultiPortSwitch  DataPortOrder=Zero-based contiguous  Inputs=1  zeroidx=on
  Index Vector1 : MultiPortSwitch  DataPortOrder=Zero-based contiguous  Inputs=1  zeroidx=on
  Relational Operator : RelationalOperator  Operator=<  OutDataTypeStr=boolean
  Switch : Switch  Criteria=u2 ~= 0
  Count : Outport
  Reg : Outport  Port=2
  Value : Outport  Port=3
  wires:
  Index Vector/1 -> Reg/1
  Constant/1 -> Index Vector/2
  Index/1 -> Index Vector/1, Index Vector1/1
  Constant2/1 -> Index Vector1/2
  Index Vector1/1 -> Value/1
  Constant4/1 -> Relational Operator/1, Switch/1
  Constant3/1 -> Relational Operator/2, Switch/3
  Relational Operator/1 -> Data Type Conversion/1
  Switch/1 -> Count/1
  Data Type Conversion/1 -> Switch/2

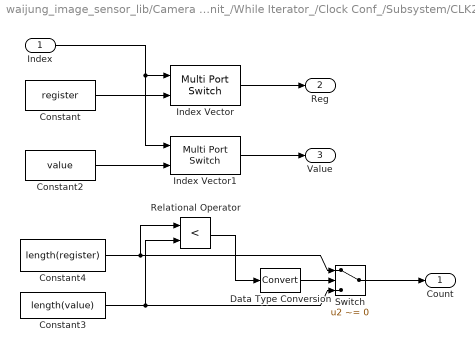
== system waijung_image_sensor_lib/Camera OV7670/Init_/While Iterator_/Clock Conf_/Subsystem/CLK24MHz_/Reg List_ ==
  Index : Inport
  Constant : Constant  Value=register
  Constant2 : Constant  Value=value
  Constant3 : Constant  Value=length(value)
  Constant4 : Constant  Value=length(register)
  Data Type Conversion : DataTypeConversion
  Index Vector : MultiPortSwitch  DataPortOrder=Zero-based contiguous  Inputs=1  zeroidx=on
  Index Vector1 : MultiPortSwitch  DataPortOrder=Zero-based contiguous  Inputs=1  zeroidx=on
  Relational Operator : RelationalOperator  Operator=<  OutDataTypeStr=boolean
  Switch : Switch  Criteria=u2 ~= 0
  Count : Outport
  Reg : Outport  Port=2
  Value : Outport  Port=3
  wires:
  Index Vector/1 -> Reg/1
  Constant/1 -> Index Vector/2
  Index/1 -> Index Vector/1, Index Vector1/1
  Constant2/1 -> Index Vector1/2
  Index Vector1/1 -> Value/1
  Constant4/1 -> Relational Operator/1, Switch/1
  Constant3/1 -> Relational Operator/2, Switch/3
  Relational Operator/1 -> Data Type Conversion/1
  Switch/1 -> Count/1
  Data Type Conversion/1 -> Switch/2

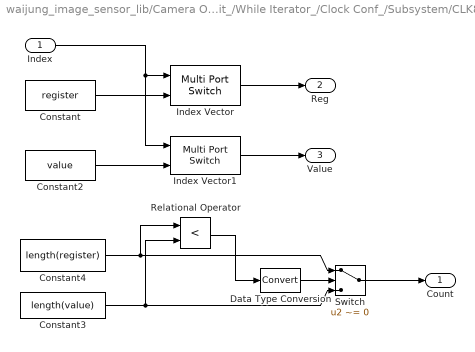
== system waijung_image_sensor_lib/Camera OV7670/Init_/While Iterator_/Clock Conf_/Subsystem/CLK8MHz_/Reg List_ ==
  Index : Inport
  Constant : Constant  Value=register
  Constant2 : Constant  Value=value
  Constant3 : Constant  Value=length(value)
  Constant4 : Constant  Value=length(register)
  Data Type Conversion : DataTypeConversion
  Index Vector : MultiPortSwitch  DataPortOrder=Zero-based contiguous  Inputs=1  zeroidx=on
  Index Vector1 : MultiPortSwitch  DataPortOrder=Zero-based contiguous  Inputs=1  zeroidx=on
  Relational Operator : RelationalOperator  Operator=<  OutDataTypeStr=boolean
  Switch : Switch  Criteria=u2 ~= 0
  Count : Outport
  Reg : Outport  Port=2
  Value : Outport  Port=3
  wires:
  Data Type Conversion/1 -> Switch/2
  Switch/1 -> Count/1
  Relational Operator/1 -> Data Type Conversion/1
  Constant3/1 -> Switch/3, Relational Operator/2
  Constant4/1 -> Switch/1, Relational Operator/1
  Index Vector1/1 -> Value/1
  Constant2/1 -> Index Vector1/2
  Index/1 -> Index Vector1/1, Index Vector/1
  Constant/1 -> Index Vector/2
  Index Vector/1 -> Reg/1

== system waijung_image_sensor_lib/Camera OV7670/Init_/While Iterator_/Picture Size_/Subsystem/Subsystem/Img120x160 ==
  Index : Inport
  Action Port : ActionPort  PropagateVarSize=During execution
  Register List : Subsystem  mask{register=uint8([58,61,140,64,18,50,23,24,25,26,3,12,62,112,113,114,115,162]), value=uint8([8,192,0,208,20,128,22,4,3,123,10,4,26,58,53,238,242,2])}
      mask prompts: register "Register Index"; value "Register Value"
      mask help:
      | Count:
      |  - Number of Register-Value pair.
      |  - Determine from lowest size, between Register and Value.
      | Reg:
      |  - Register index.
      | Value:
      |  - Data corresponding to specified register index.
  Count : Outport
  Reg : Outport  Port=2
  Value : Outport  Port=3
  wires:
  Index/1 -> Register List/1(Index)
  Register List/1(Count) -> Count/1
  Register List/2(Reg) -> Reg/1
  Register List/3(Value) -> Value/1

== system waijung_image_sensor_lib/Camera OV7670/Init_/While Iterator_/Picture Size_/Subsystem/Subsystem/Img240x320 ==
  Index : Inport
  Action Port : ActionPort  PropagateVarSize=During execution
  Register List : Subsystem  mask{register=uint8([58,61,140,64,18,50,23,24,25,26,3,12,62,112,113,114,115,162]), value=uint8([8,130,0,208,20,128,22,4,3,123,10,4,0,58,53,17,240,2])}
      mask prompts: register "Register Index"; value "Register Value"
      mask help:
      | Count:
      |  - Number of Register-Value pair.
      |  - Determine from lowest size, between Register and Value.
      | Reg:
      |  - Register index.
      | Value:
      |  - Data corresponding to specified register index.
  Count : Outport
  Reg : Outport  Port=2
  Value : Outport  Port=3
  wires:
  Register List/3(Value) -> Value/1
  Register List/2(Reg) -> Reg/1
  Register List/1(Count) -> Count/1
  Index/1 -> Register List/1(Index)

== system waijung_image_sensor_lib/Camera OV7670/Init_/While Iterator_/Picture Size_/Subsystem/Subsystem/Img480x640 ==
  Index : Inport
  Action Port : ActionPort  PropagateVarSize=During execution
  Register List : Subsystem  mask{register=uint8([58,61,140,64,18,50,23,24,25,26,3,12,62,112,113,114,115,162]), value=uint8([8,130,0,208,4,128,22,4,3,123,10,0,0,58,53,17,240,2])}
      mask prompts: register "Register Index"; value "Register Value"
      mask help:
      | Count:
      |  - Number of Register-Value pair.
      |  - Determine from lowest size, between Register and Value.
      | Reg:
      |  - Register index.
      | Value:
      |  - Data corresponding to specified register index.
  Count : Outport
  Reg : Outport  Port=2
  Value : Outport  Port=3
  wires:
  Index/1 -> Register List/1(Index)
  Register List/1(Count) -> Count/1
  Register List/2(Reg) -> Reg/1
  Register List/3(Value) -> Value/1

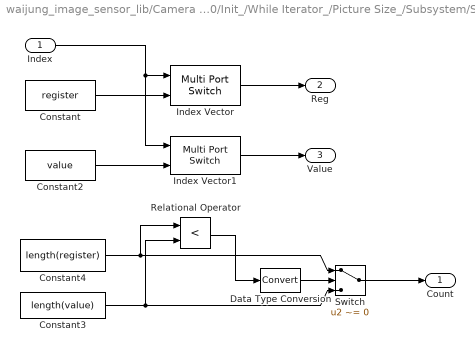
== system waijung_image_sensor_lib/Camera OV7670/Init_/While Iterator_/Picture Size_/Subsystem/Subsystem/Img120x160/Register List ==
  Index : Inport
  Constant : Constant  Value=register
  Constant2 : Constant  Value=value
  Constant3 : Constant  Value=length(value)
  Constant4 : Constant  Value=length(register)
  Data Type Conversion : DataTypeConversion
  Index Vector : MultiPortSwitch  DataPortOrder=Zero-based contiguous  Inputs=1  zeroidx=on
  Index Vector1 : MultiPortSwitch  DataPortOrder=Zero-based contiguous  Inputs=1  zeroidx=on
  Relational Operator : RelationalOperator  Operator=<  OutDataTypeStr=boolean
  Switch : Switch  Criteria=u2 ~= 0
  Count : Outport
  Reg : Outport  Port=2
  Value : Outport  Port=3
  wires:
  Data Type Conversion/1 -> Switch/2
  Switch/1 -> Count/1
  Relational Operator/1 -> Data Type Conversion/1
  Constant3/1 -> Switch/3, Relational Operator/2
  Constant4/1 -> Switch/1, Relational Operator/1
  Index Vector1/1 -> Value/1
  Constant2/1 -> Index Vector1/2
  Index/1 -> Index Vector1/1, Index Vector/1
  Constant/1 -> Index Vector/2
  Index Vector/1 -> Reg/1

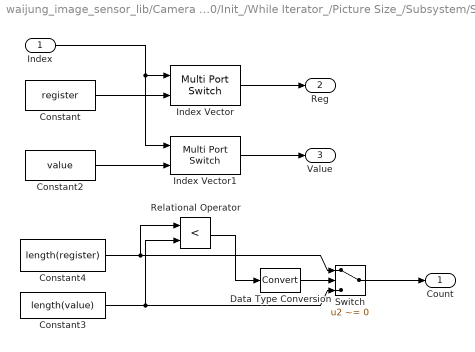
== system waijung_image_sensor_lib/Camera OV7670/Init_/While Iterator_/Picture Size_/Subsystem/Subsystem/Img240x320/Register List ==
  Index : Inport
  Constant : Constant  Value=register
  Constant2 : Constant  Value=value
  Constant3 : Constant  Value=length(value)
  Constant4 : Constant  Value=length(register)
  Data Type Conversion : DataTypeConversion
  Index Vector : MultiPortSwitch  DataPortOrder=Zero-based contiguous  Inputs=1  zeroidx=on
  Index Vector1 : MultiPortSwitch  DataPortOrder=Zero-based contiguous  Inputs=1  zeroidx=on
  Relational Operator : RelationalOperator  Operator=<  OutDataTypeStr=boolean
  Switch : Switch  Criteria=u2 ~= 0
  Count : Outport
  Reg : Outport  Port=2
  Value : Outport  Port=3
  wires:
  Index Vector/1 -> Reg/1
  Constant/1 -> Index Vector/2
  Index/1 -> Index Vector/1, Index Vector1/1
  Constant2/1 -> Index Vector1/2
  Index Vector1/1 -> Value/1
  Constant4/1 -> Relational Operator/1, Switch/1
  Constant3/1 -> Relational Operator/2, Switch/3
  Relational Operator/1 -> Data Type Conversion/1
  Switch/1 -> Count/1
  Data Type Conversion/1 -> Switch/2

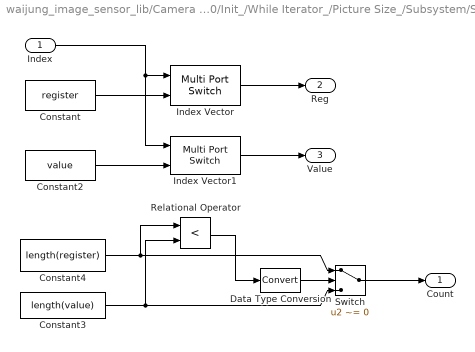
== system waijung_image_sensor_lib/Camera OV7670/Init_/While Iterator_/Picture Size_/Subsystem/Subsystem/Img480x640/Register List ==
  Index : Inport
  Constant : Constant  Value=register
  Constant2 : Constant  Value=value
  Constant3 : Constant  Value=length(value)
  Constant4 : Constant  Value=length(register)
  Data Type Conversion : DataTypeConversion
  Index Vector : MultiPortSwitch  DataPortOrder=Zero-based contiguous  Inputs=1  zeroidx=on
  Index Vector1 : MultiPortSwitch  DataPortOrder=Zero-based contiguous  Inputs=1  zeroidx=on
  Relational Operator : RelationalOperator  Operator=<  OutDataTypeStr=boolean
  Switch : Switch  Criteria=u2 ~= 0
  Count : Outport
  Reg : Outport  Port=2
  Value : Outport  Port=3
  wires:
  Data Type Conversion/1 -> Switch/2
  Switch/1 -> Count/1
  Relational Operator/1 -> Data Type Conversion/1
  Constant3/1 -> Switch/3, Relational Operator/2
  Constant4/1 -> Switch/1, Relational Operator/1
  Index Vector1/1 -> Value/1
  Constant2/1 -> Index Vector1/2
  Index/1 -> Index Vector1/1, Index Vector/1
  Constant/1 -> Index Vector/2
  Index Vector/1 -> Reg/1
